simulink model "buck48to12_physical_power_circuit"  (R2024b)
settings: Solver=ode3  StartTime=0.0  StopTime=8e-3  FixedStep=5e-7  RelTol=1e-3
values from neighbouring files (symbols this model uses):
  ctrl_mode = 2 dual voltage-current PI. Default is dual loop.']))    [build_buck48to12_physical_slx.m]
  fs = %.17g;\n"      "vref =    [run_dcdc_dual_loop_design.m]
undefined symbols (not defined in the file or in its folder): C_buck, Ki_i, Ki_v, Kp_i, Kp_v, L_buck, R_load, Vin
libraries: spsSeriesRLCBranchLib x3, spsGroundLib x1, spsDiodeLib x1, spsMosfetLib x1, spsCurrentMeasurementLib x1, spsVoltageMeasurementLib x1, simulink x1, spsDCVoltageSourceLib x1, spspowerguiLib x1
settings Model: Creator=XingTong  LastModifiedBy=XingTong

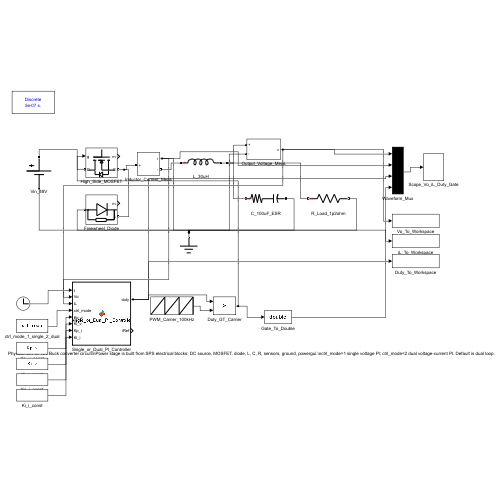
[thumbnail: Simulink's stored preview of the top-level diagram]
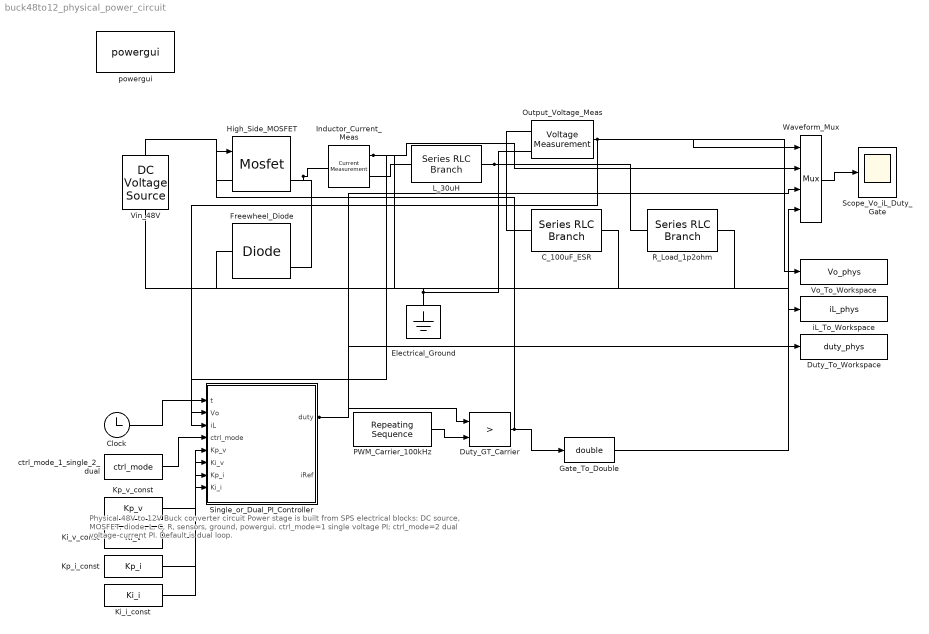
== system buck48to12_physical_power_circuit ==
  note: Physical 48V to 12V Buck converter circuit\nPower stage is built from SPS electrical blocks: DC source, MOSFET, diode, L, C, R, sensors, ground, powergui.\nctrl_mode=1 single voltage PI; ctrl_mode=2 dual voltage-current PI. Default is dual loop.
  C_100uF_ESR : spsSeriesRLCBranchLib/Series RLC Branch  LConnTagsString=__new0  RConnTagsString=__new0  BranchType=RC  Resistance=0.02  Inductance=1e-3  SetiL0=off  InitialCurrent=0  Capacitance=C_buck  Setx0=off  InitialVoltage=0  Measurements=Branch voltage
  Clock : Clock
  Duty_GT_Carrier : RelationalOperator  Operator=>  OutDataTypeStr=boolean  RndMeth=Simplest  InputSameDT=off
  Duty_To_Workspace : ToWorkspace  VariableName=duty_phys  SaveFormat=Structure With Time  SampleTime=-1
  Electrical_Ground : spsGroundLib/Ground  LConnTagsString=a
  Freewheel_Diode : spsDiodeLib/Diode  Ron=Ron_diode  Lon=0  Vf=Vf_diode  IC=0  UseSnubber=on  Rs=1e6  Cs=inf  Measurements=on
  Gate_To_Double : DataTypeConversion  OutDataTypeStr=double  SaturateOnIntegerOverflow=off  RndMeth=Floor
  High_Side_MOSFET : spsMosfetLib/Mosfet  Ron=Ron_mos  Lon=0  Rd=0.01  Vfd=0  IC=0  Rs=1e6  Cs=inf  Measurements=on
  Inductor_Current_Meas : spsCurrentMeasurementLib/Current Measurement  PhasorSimulation=off  OutputType=Complex  PSBequivalent=0
  Ki_i_const : Constant  Value=Ki_i
  Ki_v_const : Constant  Value=Ki_v
  Kp_i_const : Constant  Value=Kp_i
  Kp_v_const : Constant  Value=Kp_v
  L_30uH : spsSeriesRLCBranchLib/Series RLC Branch  LConnTagsString=__new0  RConnTagsString=__new0  BranchType=L  Resistance=0.015  Inductance=L_buck  SetiL0=off  InitialCurrent=0  Capacitance=1e-6  Setx0=off  InitialVoltage=0  Measurements=Branch current
  Output_Voltage_Meas : spsVoltageMeasurementLib/Voltage Measurement  PhasorSimulation=off  OutputType=Complex  PSBequivalent=0
  PWM_Carrier_100kHz : simulink/Sources/Repeating Sequence  rep_seq_t=[0 1/fs]  rep_seq_y=[0 1]
  R_Load_1p2ohm : spsSeriesRLCBranchLib/Series RLC Branch  LConnTagsString=__new0  RConnTagsString=__new0  BranchType=R  Resistance=R_load  Inductance=1e-3  SetiL0=off  InitialCurrent=0  Capacitance=1e-6  Setx0=off  InitialVoltage=0  Measurements=None
  Scope_Vo_iL_Duty_Gate : Scope
  Single_or_Dual_PI_Controller : MATLAB Function  TreatAsAtomicUnit=on
  Vin_48V : spsDCVoltageSourceLib/DC Voltage Source  Amplitude=Vin  Measurements=None
  Vo_To_Workspace : ToWorkspace  VariableName=Vo_phys  SaveFormat=Structure With Time  SampleTime=-1
  Waveform_Mux : Mux
  ctrl_mode_1_single_2_dual : Constant  Value=ctrl_mode
  iL_To_Workspace : ToWorkspace  VariableName=iL_phys  SaveFormat=Structure With Time  SampleTime=-1
  powergui : spspowerguiLib/powergui  Priority=1  SimulationMode=Discrete  SampleTime=5e-7  frequency=60  Iterations=50  frequencyindice=60  Pbase=100e6  ErrMax=1e-4  UnitsV=kV  UnitsW=MW  buscounter=0  FunctionMessages=off  echomessages=off  EnableUseOfTLC=off  CurrentSourceSwitches=off  DisableSnubberDevices=off  DisableRonSwitches=off  DisableVfSwitches=off  DisplayEquations=off  AutomaticDiscreteSolvers=off  SolverType=Tustin/Backward Euler (TBE)  Interpol=off  ExternalGateDelay=off  methode=off  Ts=100  x0status=blocks  SPID=on  SwTol=0  HookPort=off  NonlinearTolerance=1e-4  nMaxIteration=100  ContinueOnMaxIteration=off  RestoreLinks=warning  ResistiveCurrentMeasurement=off  Frange=[0:2:500]  Ylog=off  Xlog=on  ShowGrid=off  save=off  variable=ZData  structure=0  ZoomFFT=off  StartTime=0.0  cycles=1  DisplayStyle=1  fundamental=60  FreqAxis=off  MaxFrequency=1000  frequencyindicesteady=1  RmsSteady=1  display=off
  wires:
  Clock/1 -> Single_or_Dual_PI_Controller/1(t)
  Output_Voltage_Meas/1 -> Single_or_Dual_PI_Controller/2(Vo), Waveform_Mux/1, Vo_To_Workspace/1
  Inductor_Current_Meas/1 -> Single_or_Dual_PI_Controller/3(iL), Waveform_Mux/2, iL_To_Workspace/1
  ctrl_mode_1_single_2_dual/1 -> Single_or_Dual_PI_Controller/4(ctrl_mode)
  Kp_v_const/1 -> Single_or_Dual_PI_Controller/5(Kp_v)
  Ki_v_const/1 -> Single_or_Dual_PI_Controller/6(Ki_v)
  Kp_i_const/1 -> Single_or_Dual_PI_Controller/7(Kp_i)
  Ki_i_const/1 -> Single_or_Dual_PI_Controller/8(Ki_i)
  Single_or_Dual_PI_Controller/1(duty) -> Duty_GT_Carrier/1, Waveform_Mux/3, Duty_To_Workspace/1
  PWM_Carrier_100kHz/1 -> Duty_GT_Carrier/2
  Duty_GT_Carrier/1 -> High_Side_MOSFET/1, Gate_To_Double/1
  Gate_To_Double/1 -> Waveform_Mux/4
  Waveform_Mux/1 -> Scope_Vo_iL_Duty_Gate/1
  connections:
  Vin_48V/RConn1 -- High_Side_MOSFET/LConn1
  Inductor_Current_Meas/LConn1 -- High_Side_MOSFET/RConn1 -- Freewheel_Diode/RConn1
  Inductor_Current_Meas/RConn1 -- L_30uH/LConn1
  C_100uF_ESR/LConn1 -- L_30uH/RConn1 -- R_Load_1p2ohm/LConn1 -- Output_Voltage_Meas/LConn1
  C_100uF_ESR/RConn1 -- R_Load_1p2ohm/RConn1 -- Output_Voltage_Meas/LConn2 -- Vin_48V/LConn1 -- Electrical_Ground/LConn1 -- Freewheel_Diode/LConn1

== matlab function buck48to12_physical_power_circuit/Single_or_Dual_PI_Controller ==
  settings: updateMethod=DISCRETE  sampleTime=1e-5
  data: t input double size=1; duty output double size=1; Vo input double size=1; iL input double size=1; ctrl_mode input double size=1; Kp_v input double size=1; Ki_v input double size=1; Kp_i input double size=1; Ki_i input double size=1; iRef output double size=1
function [duty,iRef] = Single_or_Dual_PI_Controller(t,Vo,iL,ctrl_mode,Kp_v,Ki_v,Kp_i,Ki_i)
                                                                                         duty = 0; iRef = 0;                                                                       
                                                                                         persistent ev ei duty_z iref_z next_t                                                     
                                                                                         if isempty(ev)                                                                            
                                                                                             ev=0; ei=0; duty_z=0.25; iref_z=10; next_t=0;                                         
                                                                                         end                                                                                       
                                                                                         Vin_c=48; Vref_c=12; Pout_c=120; Ts=1e-5;                                                 
                                                                                         dmin=0.02; dmax=0.92; imin=0; imax=22;                                                    
                                                                                         if t >= next_t                                                                            
                                                                                             vref_now = Vref_c * min(1,t/1e-3);                                                    
                                                                                             ev_now = vref_now - Vo;                                                               
                                                                                             if ctrl_mode == 1                                                                     
                                                                                                 [duty_z, ev] = pi_lim(ev_now, ev, Kp_v, Ki_v, Ts, dmin, dmax);                    
                                                                                                 iref_z = Pout_c/Vref_c;                                                           
                                                                                             else                                                                                  
                                                                                                 [iref_z, ev] = pi_lim(ev_now, ev, Kp_v, Ki_v, Ts, imin, imax);                    
                                                                                                 ei_now = iref_z - iL;                                                             
                                                                                                 [duty_z, ei] = pi_lim(ei_now, ei, Kp_i, Ki_i, Ts, dmin, dmax);                    
                                                                                             end                                                                                   
                                                                                             next_t = next_t + Ts;                                                                 
                                                                                         end                                                                                       
                                                                                         duty = duty_z; iRef = iref_z;                                                             
                                                                                         end                                                                                       
                                                                                         function [u,integ] = pi_lim(e,integ,kp,ki,Ts,umin,umax)                                   
                                                                                         u0 = kp*e + integ;                                                                        
                                                                                         u = min(max(u0,umin),umax);                                                               
                                                                                         if (u==u0) || (u==umax && e<0) || (u==umin && e>0)                                        
                                                                                             integ = integ + ki*e*Ts;                                                              
                                                                                         end                                                                                       
                                                                                         end
